simulink model "ArucoPositionEstimation"  (R2024a)
settings: Solver=FixedStepAuto  StartTime=0.0  StopTime=inf  FixedStep=0.1  RelTol=1e-3
undefined symbols (not defined in the file): Angle, Axis, gray, VideoDirection
libraries: robotcorelib x3, eeGeneralControl x3, dspstat3 x1
settings Model: Creator=Sasha  LastModifiedBy=Sasha

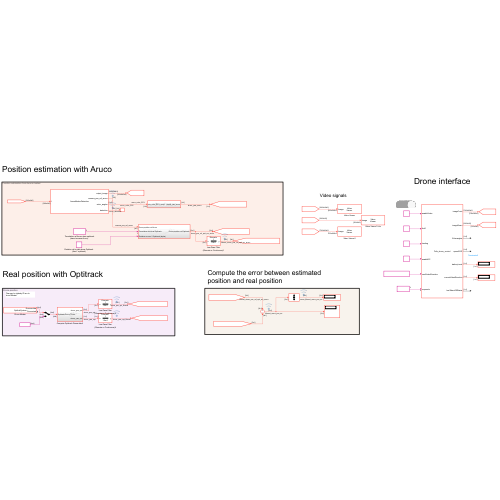
[thumbnail: Simulink's stored preview of the top-level diagram]
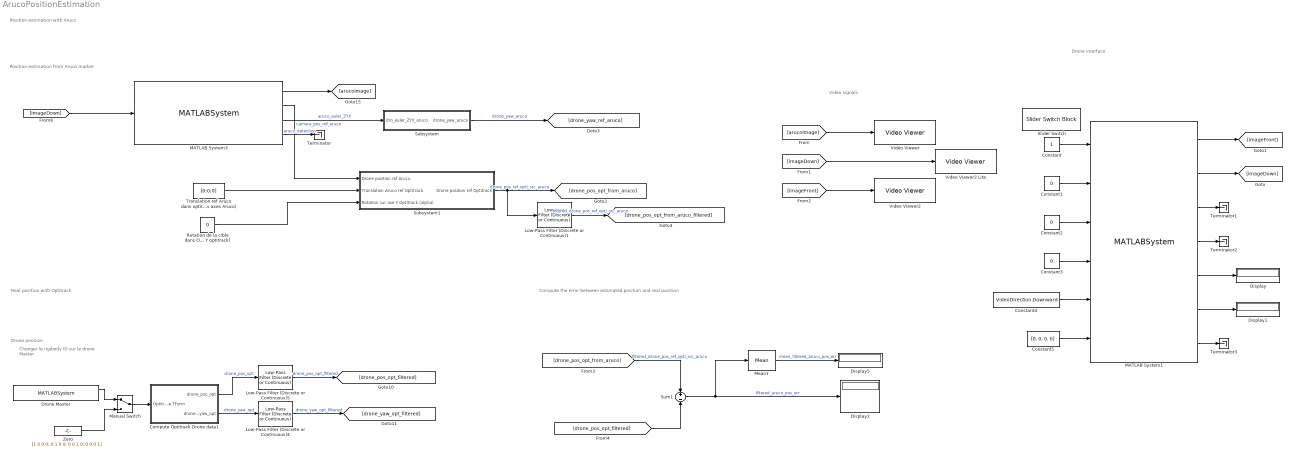
== system ArucoPositionEstimation ==
  note: Video signals
  note: Compute the error between estimated position and real position
  note: Position estimation from Aruco marker
  note: Drone position
  note: Changer le rigibody ID sur le drone Master
  note: Position estimation with Aruco
  note: Real position with Optitrack
  note: Drone interface
  Compute Optitrack Drone data1 : Subsystem
  Constant : Constant
  Constant1 : Constant  Value=0
  Constant2 : Constant  Value=0
  Constant3 : Constant  Value=0
  Constant4 : Constant  Value=VideoDirection.Downward
  Constant5 : Constant  Value=[0, 0, 0, 0]
  Display{,1..2,5} (4 alike) : Display
  Drone Master : MATLABSystem  System=OptilinkSystem  HostIP=10.147.125.15  ClientIP=10.147.125.13  RigidbodyID=4  SimulateUsing=Interpreted execution
      mask Type: OptilinkSystem
      mask Display:
      | disp('OptilinkSystem');
      | port_label('output',1,'Drones data');
      | port_label('output',2,'Connected');
  Low-Pass Filter (Discrete or Continuous)1 : eeGeneralControl/Low-Pass Filter (Discrete or Continuous)  K=1  T=1.5  B=inf  A=-inf  init_option=Inherited from block input  x0=0  Ts=-1
  Low-Pass Filter (Discrete or Continuous)4 : eeGeneralControl/Low-Pass Filter (Discrete or Continuous)  K=1  T=1.5  B=inf  A=-inf  init_option=Inherited from block input  x0=0  Ts=-1
  Low-Pass Filter (Discrete or Continuous)5 : eeGeneralControl/Low-Pass Filter (Discrete or Continuous)  K=1  T=1.5  B=inf  A=-inf  init_option=Inherited from block input  x0=0  Ts=-1
  MATLAB System1 : MATLABSystem  System=Tello_drone_control  droneIP=127.0.0.1  SimulateUsing=Interpreted execution
      mask Type: Tello_drone_control
      mask Display:
      | disp('Tello_drone_control');
      | port_label('input',1,'enableVideo');
      | port_label('input',2,'tkoff');
      | port_label('input',3,'landing');
      | port_label('input',4,'enableRC');
      | port_label('input',5,'cmdVideoDirection');
      | port_label('input',6,'rcspeeds');
      | port_label('output',1,'imageFront');
      | port_label('output',2,'imageDown');
      | port_label('output',3,'Eulerangles');
      | port_label('output',4,'speedXYZ');
      | port_label('output',5,'batteryLevel');
      | port_label('output',6,'currentVideoDirection');
      | port_label('output',7,'hasTakenOffStatus');
  MATLAB System3 : MATLABSystem  System=ArucoMarkerDetection  markerSizeInMM=150  markerFamily=DICT_4X4_250  maxMarkers=1  focalLength=[222.5, 224]  principalPoint=[156 ,116]  imageSize=[240,320]  SimulateUsing=Interpreted execution
      mask Type: ArucoMarkerDetection
      mask Display:
      | disp('ArucoMarkerDetection');
      | port_label('input',1,'I');
      | port_label('output',1,'output_image');
      | port_label('output',2,'camera_pos_ref_aruco');
      | port_label('output',3,'euler_angles');
      | port_label('output',4,'detection');
  Manual Switch : ManualSwitch
  Mean1 : dspstat3/Mean  run=off  InputProcessing=Columns as channels (frame based)  reset_popup=None  directionMode=Each row  dimension=1  roiEnable=off  roiType=Rectangles  roiPortion=Entire ROI  roiOutput=Individual statistics for each ROI  roiFlag=off  roundingMode=Floor  overflowMode=off  outputDataTypeStr=Inherit: Same as accumulator  outputMin=[]  outputMax=[]  outputLastDataTypeStr=Inherit: Same as accumulator
  Rotation de la cible dans Optitrack (Axe Y optitrack) : Constant  Value=0
  Slider Switch : SliderSwitchBlock
      settings: Values={{'Off', 'On'}, [0 1]}
  Subsystem : Subsystem
  Subsystem1 : Subsystem
  Sum1 : Sum  Inputs=+-
  Terminator{,1..3} (4 alike) : Terminator
  "Translation ref Aruco dans optitrack (dans les axes Aruco) " : Constant  Value=[0;0;0]
  Video Viewer : VideoViewer  colormapValue=gray(256)  FigPos=[754.333333333333 951.333333333333 749.333333333333 848.666666666667]
  Video Viewer2 : VideoViewer  FigPos=[974.333333333333 890 418 304]
  Video Viewer3 Lite : VideoViewer  FigPos=[1055.66666666667 642.666666666667 418 304]
  Zero : Constant  Value=[1 0 0 0; 0 1 0 0; 0 0 1 0; 0 0 0 1]  OutDataTypeStr=Inherit: Inherit via back propagation
  wires:
  MATLAB System3/2 -> Subsystem1/1(Drone position ref Aruco)  "camera_pos_ref_aruco"
  MATLAB System3/1 -> [arucoImage]
  MATLAB System1/2 -> [imageDown]
  MATLAB System1/1 -> [imageFront]
  Constant/1 -> MATLAB System1/1
  Constant1/1 -> MATLAB System1/2
  Constant2/1 -> MATLAB System1/3
  Constant3/1 -> MATLAB System1/4
  Constant4/1 -> MATLAB System1/5
  MATLAB System1/5 -> Display/1
  MATLAB System1/6 -> Display1/1
  [arucoImage] -> Video Viewer/1
  [imageFront] -> Video Viewer2/1
  [imageDown] -> Video Viewer3 Lite/1
  Low-Pass Filter (Discrete or Continuous)4/1 -> [drone_yaw_opt_filtered]  "drone_yaw_opt_filtered"
  Low-Pass Filter (Discrete or Continuous)5/1 -> [drone_pos_opt_filtered]  "drone_pos_opt_filtered"
  Manual Switch/1 -> Compute Optitrack Drone data1/1(Optitrack Drone TForm)
  Drone Master/1 -> Manual Switch/1
  Compute Optitrack Drone data1/1(drone_pos_opt) -> Low-Pass Filter (Discrete or Continuous)5/1  "drone_pos_opt"
  Zero/1 -> Manual Switch/2
  Compute Optitrack Drone data1/2(drone_yaw_opt) -> Low-Pass Filter (Discrete or Continuous)4/1  "drone_yaw_opt"
  MATLAB System3/3 -> Subsystem/1(dro_euler_ZYX_aruco)  "aruco_euler_ZYX"
  Subsystem/1(drone_yaw_aruco) -> [drone_yaw_ref_aruco]  "drone_yaw_aruco"
  [imageDown] -> MATLAB System3/1
  "Translation ref Aruco dans optitrack (dans les axes Aruco) "/1 -> Subsystem1/2(Translation Aruco ref Optitrack)
  Rotation de la cible dans Optitrack (Axe Y optitrack)/1 -> Subsystem1/3(Rotation sur axe Y Optitrack (alpha))
  [drone_pos_opt_from_aruco] -> Sum1/1  "filtered_drone_pos_ref_opti_src_aruco"
  Sum1/1 -> Mean1/1, Display2/1  "filtered_aruco_pos_err"
  Mean1/1 -> Display5/1  "mean_filtered_aruco_pos_err"
  MATLAB System3/4 -> Terminator/1  "aruco_detection"
  Subsystem1/1(Drone position ref Optitrack) -> Low-Pass Filter (Discrete or Continuous)1/1, [drone_pos_opt_from_aruco]  "drone_pos_ref_opti_src_aruco"
  [drone_pos_opt_filtered] -> Sum1/2
  Low-Pass Filter (Discrete or Continuous)1/1 -> [drone_pos_opt_from_aruco_filtered]  "filtered_drone_pos_ref_opti_src_aruco"
  Constant5/1 -> MATLAB System1/6
  MATLAB System1/3 -> Terminator1/1
  MATLAB System1/4 -> Terminator2/1
  MATLAB System1/7 -> Terminator3/1

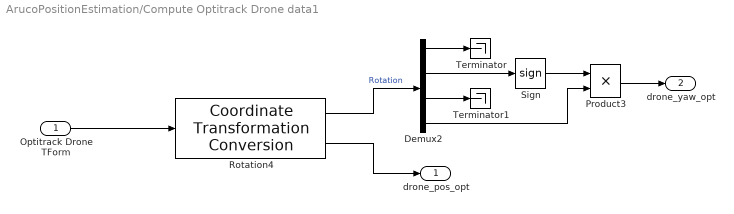
== system ArucoPositionEstimation/Compute Optitrack Drone data1 ==
  Optitrack Drone TForm : Inport
  Demux2 : Demux
  Product3 : Product
  Rotation4 : robotcorelib/Coordinate Transformation Conversion  InputRepresentation=Homogeneous Transformation  InputEulerSequence=XYZ  ShowTrVecInputPort=on  OutputRepresentation=Axis-Angle  OutputEulerSequence=XYZ  ShowTrVecOutputPort=on  SimulateUsing=Code generation
      settings: LibrarySourceBlock=uavutilslib/Coordinate Transformation Conversion
  Sign : Signum
  Terminator : Terminator
  Terminator1 : Terminator
  drone_pos_opt : Outport
  drone_yaw_opt : Outport  Port=2
  wires:
  Rotation4/2 -> drone_pos_opt/1
  Demux2/4 -> Product3/2
  Rotation4/1 -> Demux2/1  "Rotation"
  Sign/1 -> Product3/1
  Demux2/2 -> Sign/1
  Product3/1 -> drone_yaw_opt/1
  Optitrack Drone TForm/1 -> Rotation4/1
  Demux2/3 -> Terminator1/1
  Demux2/1 -> Terminator/1

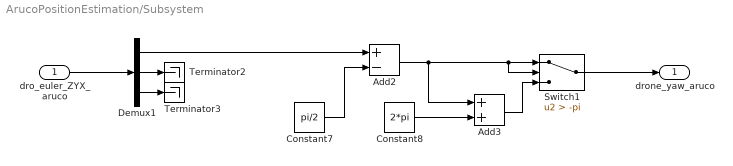
== system ArucoPositionEstimation/Subsystem ==
  dro_euler_ZYX_aruco : Inport
  Add2 : Sum  Inputs=+-
  Add3 : Sum
  Constant7 : Constant  Value=pi/2
  Constant8 : Constant  Value=2*pi
  Demux1 : Demux  Outputs=3
  Switch1 : Switch  Criteria=u2 > Threshold  Threshold=-pi  SaturateOnIntegerOverflow=off  InputSameDT=off
  Terminator2 : Terminator
  Terminator3 : Terminator
  drone_yaw_aruco : Outport
  wires:
  dro_euler_ZYX_aruco/1 -> Demux1/1
  Add2/1 -> Add3/1, Switch1/2, Switch1/1
  Demux1/3 -> Terminator3/1
  Constant8/1 -> Add3/2
  Demux1/1 -> Add2/1
  Add3/1 -> Switch1/3
  Constant7/1 -> Add2/2
  Demux1/2 -> Terminator2/1
  Switch1/1 -> drone_yaw_aruco/1

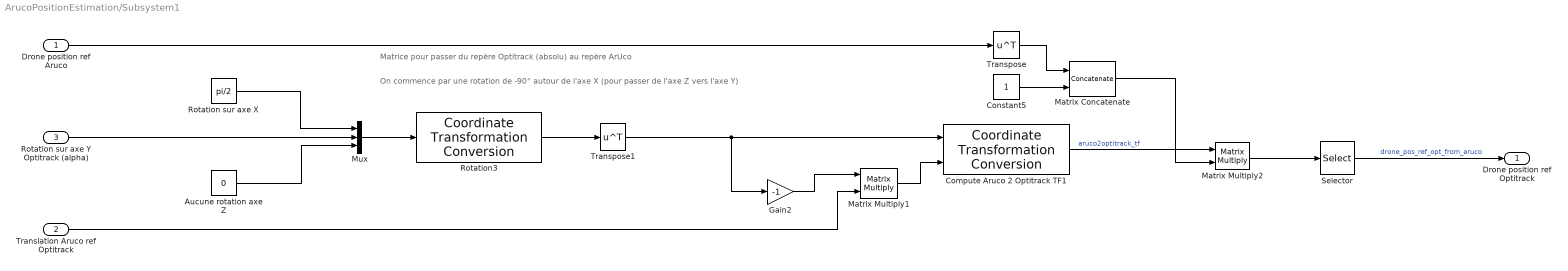
== system ArucoPositionEstimation/Subsystem1 ==
  note: Matrice pour passer du repère Optitrack (absolu) au repère ArUco
  note: On commence par une rotation de -90° autour de l'axe X (pour passer de l'axe Z vers l'axe Y)
  Drone position ref Aruco : Inport
  Translation Aruco ref Optitrack : Inport  Port=2
  Rotation sur axe Y Optitrack (alpha) : Inport  Port=3
  Aucune rotation axe Z : Constant  Value=0
  Compute Aruco 2 Optitrack TF1 : robotcorelib/Coordinate Transformation Conversion  InputRepresentation=Rotation Matrix  InputEulerSequence=XYZ  ShowTrVecInputPort=on  OutputRepresentation=Homogeneous Transformation  OutputEulerSequence=XYZ  ShowTrVecOutputPort=on  SimulateUsing=Code generation
      settings: LibrarySourceBlock=uavutilslib/Coordinate Transformation Conversion
  Constant5 : Constant
  Gain2 : Gain  Gain=-1
  Matrix Concatenate : Concatenate  ConcatenateDimension=2
  Matrix Multiply1 : Product  Multiplication=Matrix(*)
  Matrix Multiply2 : Product  Multiplication=Matrix(*)
  Mux : Mux  Inputs=3
  Rotation sur axe X : Constant  Value=pi/2
  Rotation3 : robotcorelib/Coordinate Transformation Conversion  InputRepresentation=Euler Angles  InputEulerSequence=XYZ  ShowTrVecInputPort=on  OutputRepresentation=Rotation Matrix  OutputEulerSequence=XYZ  ShowTrVecOutputPort=on  SimulateUsing=Code generation
      settings: LibrarySourceBlock=uavutilslib/Coordinate Transformation Conversion
  Selector : Selector  InputPortWidth=4  IndexOptions=Index vector (dialog)  Indices=[1 2 3]  OutputSizes=1
  Transpose : Math  Operator=transpose
  Transpose1 : Math  Operator=transpose
  Drone position ref Optitrack : Outport
  wires:
  Rotation sur axe Y Optitrack (alpha)/1 -> Mux/2
  Transpose/1 -> Matrix Concatenate/1
  Mux/1 -> Rotation3/1
  Constant5/1 -> Matrix Concatenate/2
  Gain2/1 -> Matrix Multiply1/1
  Rotation3/1 -> Transpose1/1
  Matrix Multiply1/1 -> Compute Aruco 2 Optitrack TF1/2
  Rotation sur axe X/1 -> Mux/1
  Transpose1/1 -> Gain2/1, Compute Aruco 2 Optitrack TF1/1
  Matrix Concatenate/1 -> Matrix Multiply2/2
  Aucune rotation axe Z/1 -> Mux/3
  Compute Aruco 2 Optitrack TF1/1 -> Matrix Multiply2/1  "aruco2optitrack_tf"
  Matrix Multiply2/1 -> Selector/1
  Selector/1 -> Drone position ref Optitrack/1  "drone_pos_ref_opt_from_aruco"
  Drone position ref Aruco/1 -> Transpose/1
  Translation Aruco ref Optitrack/1 -> Matrix Multiply1/2
